simulink model "soft_thresholding_hdl"  (R2021a)
settings: Solver=FixedStepDiscrete  StartTime=0.0  StopTime=10.0  RelTol=1e-3
undefined symbols (not defined in the file): lambda2
settings Model: DataTypeOverride=Off  Creator=Bhea Vasquez  LastModifiedBy=Bhea Vasquez
settings OptimizationCC: BlockReduction=off  ConditionallyExecuteInputs=off  DefaultParameterBehavior=Inlined
settings DebuggingCC: AlgebraicLoopMsg=error  SingleTaskRateTransMsg=error
settings HardwareCC: ProdBitPerPointer=32  ProdBitPerSizeT=32  ProdBitPerPtrDiffT=32  ProdLargestAtomicFloat=None  ProdIntDivRoundTo=Undefined  ProdEndianess=Unspecified  ProdWordSize=32  ProdHWDeviceType=ASIC/FPGA->ASIC/FPGA  TargetBitPerPointer=64  TargetBitPerSizeT=64  TargetBitPerPtrDiffT=64  TargetLongLongMode=on  TargetIntDivRoundTo=Zero  TargetEndianess=LittleEndian  TargetWordSize=64  TargetHWDeviceType=Custom Processor->MATLAB Host Computer  ProdEqTarget=off

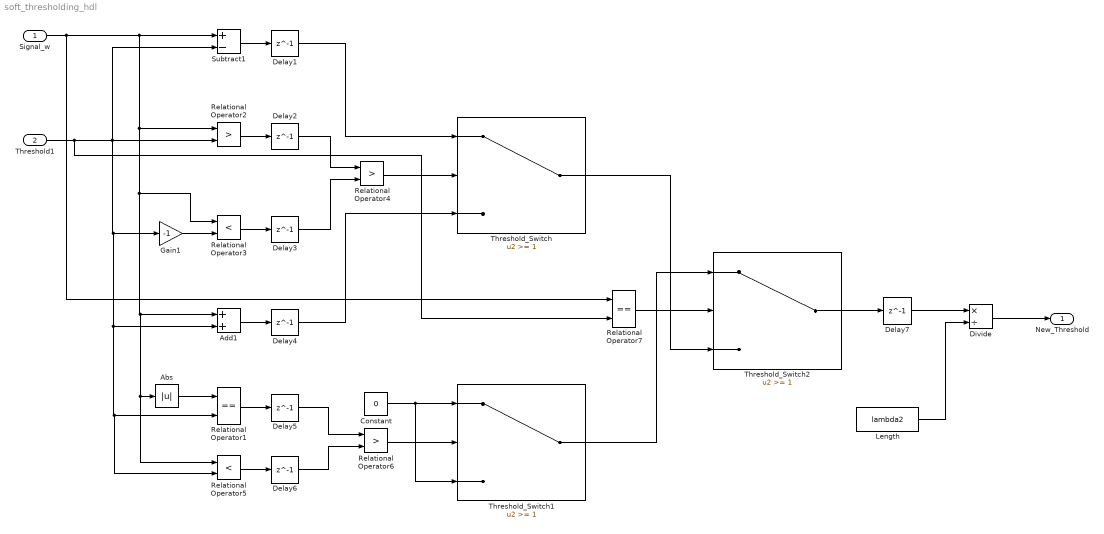
== system soft_thresholding_hdl ==
  Signal_w : Inport  OutDataTypeStr=fixdt(1,16,12)
  Threshold1 : Inport  Port=2  OutDataTypeStr=fixdt(1,16,12)
  Abs : Abs  OutDataTypeStr=fixdt(1,16,12)
  Add1 : Sum  AccumDataTypeStr=fixdt(1,16,24)  OutDataTypeStr=fixdt(1,16,24)
  Constant : Constant  Value=0  OutDataTypeStr=fixdt(1,16,12)  SampleTime=-1
  Delay{1..7} (7 alike) : Delay  DelayLength=1
  Divide : Product  Inputs=*/  OutDataTypeStr=fixdt(1,16,12)  RndMeth=Simplest  SaturateOnIntegerOverflow=on
  Gain1 : Gain  Gain=-1  ParamDataTypeStr=fixdt(1,16,12)  OutMin=-1  OutMax=-0.99  OutDataTypeStr=fixdt(1,16,12)
  Length : Constant  Value=lambda2  OutDataTypeStr=fixdt(1,16,12)  SampleTime=-1
  Relational Operator1 : RelationalOperator  Operator===  OutDataTypeStr=fixdt(1,16,12)  RndMeth=Simplest
  Relational Operator2 : RelationalOperator  Operator=>  OutDataTypeStr=fixdt(1,16,12)  RndMeth=Simplest
  Relational Operator3 : RelationalOperator  Operator=<  OutDataTypeStr=fixdt(1,16,12)  RndMeth=Simplest
  Relational Operator4 : RelationalOperator  Operator=>  OutDataTypeStr=fixdt(1,16,12)  RndMeth=Simplest
  Relational Operator5 : RelationalOperator  Operator=<  OutDataTypeStr=fixdt(1,16,12)  RndMeth=Simplest
  Relational Operator6 : RelationalOperator  Operator=>  OutDataTypeStr=fixdt(1,16,12)  RndMeth=Simplest
  Relational Operator7 : RelationalOperator  Operator===  OutDataTypeStr=fixdt(1,16,12)  RndMeth=Simplest
  Subtract1 : Sum  Inputs=+-  AccumDataTypeStr=fixdt(1,16,24)  OutDataTypeStr=fixdt(1,16,24)
  Threshold_Switch : Switch  Threshold=1  OutDataTypeStr=fixdt(1,16,12)
  Threshold_Switch1 : Switch  Threshold=1  OutDataTypeStr=fixdt(1,16,12)
  Threshold_Switch2 : Switch  Threshold=1  OutDataTypeStr=fixdt(1,16,12)
  New_Threshold : Outport  OutDataTypeStr=fixdt(1,16,12)
  wires:
  Delay1/1 -> Threshold_Switch/1
  Signal_w/1 -> Subtract1/1, Relational Operator2/1, Relational Operator5/1, Abs/1, Add1/1, Relational Operator3/1, Relational Operator7/1
  Relational Operator1/1 -> Delay5/1
  Delay2/1 -> Relational Operator4/1
  Delay5/1 -> Relational Operator6/1
  Subtract1/1 -> Delay1/1
  Threshold_Switch2/1 -> Delay7/1
  Delay4/1 -> Threshold_Switch/3
  Delay6/1 -> Relational Operator6/2
  Relational Operator7/1 -> Threshold_Switch2/2
  Relational Operator4/1 -> Threshold_Switch/2
  Delay7/1 -> Divide/1
  Gain1/1 -> Relational Operator3/2
  Relational Operator6/1 -> Threshold_Switch1/2
  Constant/1 -> Threshold_Switch1/3, Threshold_Switch1/1
  Add1/1 -> Delay4/1
  Relational Operator5/1 -> Delay6/1
  Abs/1 -> Relational Operator1/1
  Threshold1/1 -> Relational Operator2/2, Subtract1/2, Relational Operator5/2, Relational Operator1/2, Add1/2, Gain1/1, Relational Operator7/2
  Divide/1 -> New_Threshold/1
  Threshold_Switch1/1 -> Threshold_Switch2/1
  Relational Operator3/1 -> Delay3/1
  Length/1 -> Divide/2
  Relational Operator2/1 -> Delay2/1
  Delay3/1 -> Relational Operator4/2
  Threshold_Switch/1 -> Threshold_Switch2/3
